simulink model "vehicle_hostmodel_2022b_v10"  (R2024b)
settings: Solver=ode4  StartTime=0.0  StopTime=inf  FixedStep=0.01  MaxStep=0.05  RelTol=1e-3
PreLoadFcn:
  | load("FInalGraph.mat")
model workspace (MAT data in the model file):
  G_final : digraph (value not decoded)
values from neighbouring files (symbols this model uses):
  ActorID = 0    [HelperSpeedActionAdapter.m]
  D = cross(B-A,C-A)    [HelperCalculateEgoRefPathInfo.m]
  L = zeros(N,1)    [HelperCalculateEgoRefPathInfo.m]
  psi_o = -1.185    [sensor.m]
  R = NaN(N,1)    [HelperCalculateEgoRefPathInfo.m]
  SceneInfo = [-32.1351766513 25.1612903226 -74.2242703533 -71.4592933948 -32.2887864823 26.2365591398 26.8509984639 27.0046082949 -32.7496159754 -72.380952381 -49.846390169 -49.3855606759 ... (30 elements, 10x3)]    [SceneLabels.mat]
  Ts = 0.05    [sensor.m]
undefined symbols (not defined in the file or in its folder): Acceleration, AngularVelocity, barrier_1, barrier_2, barrier_3, curvature, DefaultGear, DEND_B, DEND_S, DEND_T, direction, DiscIntNeverNeededParam, driving, finalint, goal1_coordinates, goal2_coordinates, goal3_coordinates, gradbp, latlongcoordinates, LF, LR, matlabshared, MAX_BRAKE, MAX_STEER, MAX_TORQUE, MCAR, MIN_BRAKE, MIN_STEER, MIN_TORQUE, NUMD_B, NUMD_S, NUMD_T, Pitch, Position, Roll, RRdamp, session, sigbuilder_block, STEER_RATIO, stopSign_ID, Tdead, thetaRefs, TL_ID, TrackWidth, ts, Vdead, Velocity, WB, xRef2s, Yaw, yRef2s
libraries: simulink x12, drivingscenarioandsensors x8, simulink_extras x5, drivingvehiclecontroller x2, trackingutilitieslib x2, robotalgslib x1, mpcadaslib x1, slpidlib x1, drivinglib x1, mpclib x1, autolibshared x1, vehdynlibviscommon x1
(part 1 of 4)
settings Model: SILPILSystemUnderTest=refmodels  Creator=akshran  LastModifiedBy=karto
settings DataIOCC: SignalLogging=off
settings OptimizationCC: ReuseModelBlockBuffer=off  ZeroExternalMemoryAtStartup=off  ZeroInternalMemoryAtStartup=off
settings DebuggingCC: UnconnectedInputMsg=warning  UnconnectedOutputMsg=warning  UnconnectedLineMsg=warning  UnderSpecifiedDimensionMsg=warning
settings HardwareCC: ProdBitPerLong=64  ProdHWDeviceType=Apple->ARM64
settings ModelReferenceCC: EnableRefExpFcnMdlSchedulingChecks=on
settings RTWCC: GenCodeOnly=on  TargetLang=C++  GPUComputeCapability=3.5  DLArmComputeVersion=19.05
settings GRTTargetCC: TargetLangStandard=C++11 (ISO)  MatFileLogging=off  CodeInterfacePackaging=C++ class

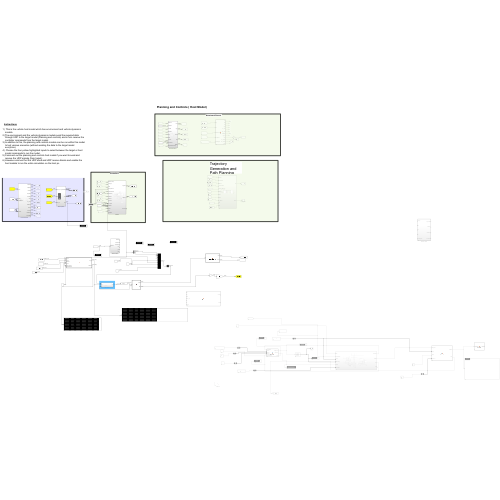
[thumbnail: Simulink's stored preview of the top-level diagram]
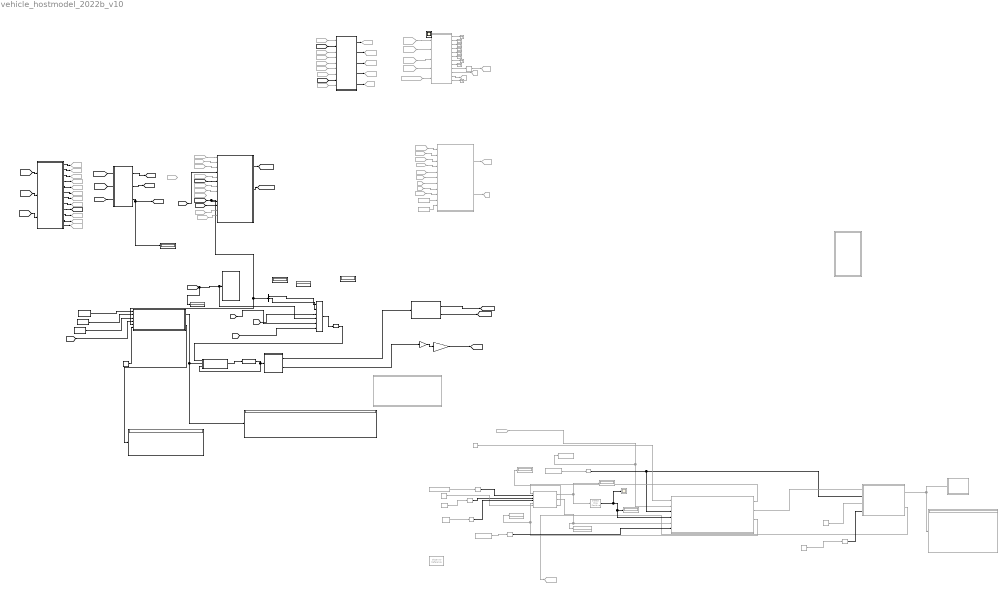
== system vehicle_hostmodel_2022b_v10 ==
  note: Trajectory Generation and Path Planning
  note: Trajectory Generation
  note: Behavioural Planner
  note: Instructions
      |
      | This is the vehicle host model which has environment and vehicle dynamics models.
      | The environment and the vehicle dynamics models send the required data through UDP to the target model (Planning and controls) and in turn receive the controller commands from the target model.
      | In addition to this, the planning and controls module can be run within this model to test various scenarios (without sending the data to the target model everytime).
      | Choose the four yellow highlighted inputs to select between the target or host model commands to run the model.
      | Comment out the planning and controls host model if you want to send and receive the UDP signals (from target).
      | Likewise comment out the UDP send and UDP receive blocks and enable the host models to run the entire simulation on the host pc.
  note: Environment & Vehicle Dynamics(Common Model)
  note: Planning and Controls ( Host Model)
  note: Controllers
  Behavioural Planner : Subsystem
  Constant : Constant  Value=xRef2s
  Constant1 : Constant  Commented=on  Value=latlongcoordinates
  Constant10 : Constant  Value=yRef2s
  Constant11 : Constant  Value=curvature
  Constant12 : Constant  Value=10
  Constant2 : Constant  Commented=on  Value=[latlongcoordinates(1,1) latlongcoordinates(1,2) 234]
  Constant3 : Constant  Commented=on  Value=barrier_1
  Constant4 : Constant  Commented=on  Value=40
  Constant5 : Constant  Commented=on  Value=234
  Constant6 : Constant  Commented=on  Value=goal1_coordinates
  Constant7 : Constant  Commented=on  Value=barrier_2
  Constant8 : Constant  Commented=on  Value=goal3_coordinates
  Constant9 : Constant  Commented=on  Value=barrier_3
  Controllers : Subsystem
  Demux : Demux  Outputs=3
  Detect Rise Positive : simulink/Logic and Bit Operations/Detect Rise Positive  Commented=through  vinit=0  OutDataTypeStr=boolean
  Display{,1..5} (6 alike) : Display  Commented=on
  Display{7..12,14} (7 alike) : Display
  Environment & Data : Subsystem
  From Workspace : FromWorkspace  Commented=on  VariableName=xRef2
  From Workspace1 : FromWorkspace  Commented=on  VariableName=yRef2
  From1 : From  Commented=on  GotoTag=CurrPos  TagVisibility=global
  From19 : From  Commented=on  GotoTag=obj_ahead  TagVisibility=global
  From21 : From  Commented=on  GotoTag=sceneID  TagVisibility=global
  From22 : From  Commented=on  GotoTag=objDist  TagVisibility=global
  From23 : From  Commented=on  GotoTag=D2S  TagVisibility=global
  From24 : From  Commented=on  GotoTag=SDist  TagVisibility=global
  From25 : From  Commented=on  GotoTag=TL_poses  TagVisibility=global
  From27 : From  Commented=on  GotoTag=obj_rel_vel  TagVisibility=global
  From28 : From  Commented=on  GotoTag=obj_rel_vel  TagVisibility=global
  From29 : From  Commented=on  GotoTag=RelDistMin  TagVisibility=global
  From31 : From  Commented=on  GotoTag=RefPoses
  From32 : From  Commented=on  GotoTag=direction
  From33 : From  Commented=on  GotoTag=curvature
  From36 : From  Commented=on  GotoTag=actorsInfo  TagVisibility=global
  From37 : From  Commented=on  GotoTag=ego_states  TagVisibility=global
  From38 : From  Commented=on  GotoTag=LaneBounds  TagVisibility=global
  From39 : From  Commented=on  GotoTag=RoadSpeed  TagVisibility=global
  From40 : From  Commented=on  GotoTag=CurrPos  TagVisibility=global
  From41 : From  Commented=on  GotoTag=curvature
  From42 : From  Commented=on  GotoTag=ego_vel  TagVisibility=global
  From43 : From  Commented=on  GotoTag=PositionMIO  TagVisibility=global
  From44 : From  Commented=on  GotoTag=obj_rel_vel  TagVisibility=global
  From45 : From  Commented=on  GotoTag=flagLC  TagVisibility=global
  From46 : From  Commented=on  GotoTag=laneL  TagVisibility=global
  From47 : From  Commented=on  GotoTag=desiredV  TagVisibility=global
  From48 : From  Commented=on  GotoTag=desiredV  TagVisibility=global
  From49 : From  Commented=on  GotoTag=laneR  TagVisibility=global
  From52 : From  Commented=on  GotoTag=Brake  TagVisibility=global
  From54 : From  Commented=on  GotoTag=Tgap  TagVisibility=global
  From55 : From  Commented=on  GotoTag=flagACC  TagVisibility=global
  From56 : From  Commented=on  GotoTag=LCinProgress  TagVisibility=global
  From58 : From  Commented=on  GotoTag=Acc  TagVisibility=global
  Gain1 : Gain  Gain=1/STEER_RATIO
  Gain2 : Gain  Gain=180/pi
  Goto1 : Goto  Commented=on  GotoTag=dest1  TagVisibility=global
  Goto10 : Goto  Commented=on  GotoTag=objDist  TagVisibility=global
  Goto11 : Goto  Commented=on  GotoTag=SDist  TagVisibility=global
  Goto12 : Goto  Commented=on  GotoTag=D2S  TagVisibility=global
  Goto13 : Goto  Commented=on  GotoTag=TL_poses  TagVisibility=global
  Goto16 : Goto  Commented=on  GotoTag=actorsInfo  TagVisibility=global
  Goto17 : Goto  Commented=on  GotoTag=RelDistMin  TagVisibility=global
  Goto21 : Goto  Commented=on  GotoTag=waypoints  TagVisibility=global
  Goto24 : Goto  Commented=on  GotoTag=trans_host  TagVisibility=global
  Goto25 : Goto  Commented=on  GotoTag=LaneBounds  TagVisibility=global
  Goto26 : Goto  Commented=on  GotoTag=PositionMIO  TagVisibility=global
  Goto27 : Goto  Commented=on  GotoTag=flagLC  TagVisibility=global
  Goto28 : Goto  Commented=on  GotoTag=desiredV  TagVisibility=global
  Goto29 : Goto  Commented=on  GotoTag=laneL  TagVisibility=global
  Goto30 : Goto  Commented=on  GotoTag=laneR  TagVisibility=global
  Goto32 : Goto  Commented=on  GotoTag=Brake  TagVisibility=global
  Goto33 : Goto  Commented=on  GotoTag=Tgap  TagVisibility=global
  Goto34 : Goto  Commented=on  GotoTag=flagACC  TagVisibility=global
  Goto6 : Goto  Commented=on  GotoTag=obj_ahead  TagVisibility=global
  Goto8 : Goto  Commented=on  GotoTag=obj_rel_vel  TagVisibility=global
  Goto9 : Goto  Commented=on  GotoTag=sceneID  TagVisibility=global
  LC_Progress : Goto  Commented=on  GotoTag=LC_ACC  TagVisibility=global
  MATLAB Function : MATLAB Function  Commented=on  TreatAsAtomicUnit=on
  MATLAB Function1 : MATLAB Function  Commented=through  TreatAsAtomicUnit=on
  MATLAB Function2 : MATLAB Function  TreatAsAtomicUnit=on
  MATLAB Function3 : MATLAB Function  Commented=on  TreatAsAtomicUnit=on
  MATLAB Function4 : MATLAB Function  Commented=on  TreatAsAtomicUnit=on
  MATLAB Function5 : MATLAB Function  Commented=on  TreatAsAtomicUnit=on
  MATLAB Function6 : MATLAB Function  TreatAsAtomicUnit=on
  MATLAB Function7 : MATLAB Function  TreatAsAtomicUnit=on
  Mux : Mux  Inputs=6
  NOT : Logic  Commented=on  Operator=NOT  IconShape=distinctive  AllPortsSameDT=off  OutDataTypeStr=boolean
  Observer : ObserverReference  Commented=on  ObserverModelName=vehicle_hostmodel_2022b_v10_Observer1
  Reference Data : Subsystem  VariantControl=Stanley
  Reference Data1 : Subsystem  Commented=on  TreatAsAtomicUnit=on  VariantControl=Stanley
  Reshape{,1..4,6} (6 alike) : Reshape  Commented=through  OutputDimensionality=Row vector (2-D)
  Reshape5 : Reshape  OutputDimensionality=Column vector (2-D)
  Scope2 : Scope  Commented=on
  Signal Specification : SignalSpecification  Dimensions=[2 1]
  Subsystem : Subsystem  Commented=on
  Subsystem2 : Subsystem  Commented=on
  Subsystem3 : Subsystem
  Terminator{,1..8} (9 alike) : Terminator  Commented=on
  To Workspace : ToWorkspace  Commented=on  VariableName=VehiclePos  SaveFormat=Timeseries  SampleTime=-1
  Vehicle Dynamics : Subsystem
  Scope : Scope
  Scope1 : Scope
  tag scope: CurrPos=global, MPCaccel=global, MPCdecel=global, VehInfo=global, brake_host=global, ego_states=global, ego_vel=global, steer_host=global, torque_host=global
  wires:
  Controllers/1(TorgueCm) -> [torque_host]
  Environment & Data/1(ObjAhead) -> Goto6/1
  Environment & Data/2(ObjRelVel) -> Goto8/1
  Environment & Data/3(SceneID) -> Goto9/1
  Environment & Data/4(ObjectDist) -> Goto10/1
  Environment & Data/6(SDist) -> Goto11/1
  Environment & Data/5(SceneDist) -> Goto12/1
  Environment & Data/7(TL_poses) -> Goto13/1
  Vehicle Dynamics/1(EgoVehStates) -> [ego_states]
  Vehicle Dynamics/3(xdot) -> Display8/1, [ego_vel]
  Environment & Data/8(RelDistmin) -> Goto17/1
  Vehicle Dynamics/2(Info) -> [VehInfo]
  [torque_host] -> Vehicle Dynamics/1(torque_cm)
  [brake_host] -> Vehicle Dynamics/2(brake_cm)
  [steer_host] -> Vehicle Dynamics/3(steer_cm)
  [trans_host] -> Environment & Data/1(Trans)
  [ego_states] -> Environment & Data/2(EgoVehStates)
  From28/1 -> Controllers/1(Relative velocity)
  From29/1 -> Controllers/5(Relative distance)
  [ego_vel] -> Controllers/6(CurrVelocity)
  From31/1 -> Controllers/7(RefPoses)
  From32/1 -> Controllers/8(Direction)
  [CurrPos] -> MATLAB Function2/5(current_position), Demux/1, Controllers/10(curr poses)
  [VehInfo] -> Environment & Data/3(VehFdbk)
  Environment & Data/9(CurrPos) -> [CurrPos]
  Environment & Data/10(actorsinfo) -> Goto16/1
  From37/1 -> MATLAB Function/1(ego)
  From36/1 -> MATLAB Function/2(act)
  Environment & Data/11(LaneBounds) -> Goto25/1
  From38/1 -> MATLAB Function/3(LaneBounds)
  From39/1 -> MATLAB Function/4(RoadSpeed)
  MATLAB Function/9(stay) -> NOT/1
  MATLAB Function/10(LL_Change) -> Goto29/1
  MATLAB Function/11(RL_Change) -> Goto30/1
  Environment & Data/12(PositionMIO) -> Goto26/1
  NOT/1 -> Goto27/1
  From54/1 -> Controllers/2(Time gap)
  From55/1 -> Controllers/3(ACC)
  From56/1 -> MATLAB Function/5(LCinProgress)
  [VehInfo] -> Controllers/11(VehFdbk)
  Controllers/2(BrakeCm) -> [brake_host]
  From45/1 -> Subsystem/1(function)
  From40/1 -> Subsystem/2(CurrentPose)
  From43/1 -> Subsystem/3(MIOPos)
  From41/1 -> Subsystem/4(Road Curvature)
  From42/1 -> Subsystem/5(Velocity_Initial_Ego)
  From44/1 -> Subsystem/6(MIOVel)
  From48/1 -> Subsystem/9(V_desired)
  Subsystem/2(check) -> LC_Progress/1
  From19/1 -> Behavioural Planner/1(ObjAhead)
  [ego_vel] -> Behavioural Planner/2(EgoSpeed)
  From21/1 -> Behavioural Planner/3(SceneID)
  From22/1 -> Behavioural Planner/4(ObjectDist)
  From23/1 -> Behavioural Planner/5(D2S)
  From24/1 -> Behavioural Planner/6(SDist)
  From25/1 -> Behavioural Planner/7(TLposes)
  [CurrPos] -> Behavioural Planner/8(CurrentPose)
  From27/1 -> Behavioural Planner/9(Object Relative Velocity)
  Behavioural Planner/1(Trans) -> Goto24/1
  Behavioural Planner/2(Tgap) -> Goto33/1
  Behavioural Planner/3(VelCmd) -> Goto28/1
  Behavioural Planner/4(ACC) -> Goto34/1
  Behavioural Planner/5(Braking) -> Goto32/1
  From52/1 -> Controllers/12(Brake)
  From58/1 -> Controllers/13(Acc)
  Subsystem/1(out) -> Goto21/1
  From46/1 -> Subsystem/7(laneL)
  From49/1 -> Subsystem/8(laneR)
  From Workspace/1 -> Subsystem/10(xref)
  From Workspace1/1 -> Subsystem/11(yref)
  MATLAB Function/1(ttc) -> Terminator/1
  MATLAB Function/2(dist) -> Terminator1/1
  MATLAB Function/3(left) -> Terminator2/1
  MATLAB Function/4(right) -> Terminator3/1
  MATLAB Function/5(LL_avail) -> Terminator4/1
  MATLAB Function/6(RL_avail) -> Terminator5/1
  MATLAB Function/7(tend2stay) -> Terminator6/1
  MATLAB Function/8(ego_vel) -> Terminator7/1
  MATLAB Function/12(y_lane) -> Terminator8/1
  [RoadSpeed] -> Controllers/4(velocity desired)
  From1/1 -> Subsystem2/2(CurrentPose), To Workspace/1
  MATLAB Function3/2(outbarrier) -> Display1/1, Subsystem2/5(barrier)
  MATLAB Function4/1(WPENU) -> Display/1, MATLAB Function1/1(EgoWayPts)
  MATLAB Function4/2(dest) -> Goto1/1
  Constant3/1 -> Reshape1/1
  Constant7/1 -> Reshape3/1
  Reshape3/1 -> MATLAB Function3/3(barrier2)
  Reshape/1 -> MATLAB Function4/2(origin), Subsystem2/3(origin)
  Constant4/1 -> MATLAB Function3/6(distanceBarrier)
  Subsystem2/3(flag) -> MATLAB Function3/5(ChkPointFlag), Display2/1
  Reshape1/1 -> MATLAB Function3/2(barrier1)
  Subsystem2/1(CurrPosLL) -> MATLAB Function3/1(CurrentPose)
  Constant1/1 -> Subsystem2/1(WP)
  MATLAB Function3/1(FlagBarrier) -> Detect Rise Positive/1, Display3/1
  Constant5/1 -> MATLAB Function4/3(height)
  Constant2/1 -> Reshape/1
  Reshape4/1 -> MATLAB Function4/4(goalcoord)
  Subsystem2/2(OutWP) -> MATLAB Function4/1(Waypoints)
  Reshape6/1 -> MATLAB Function3/4(barrier3)
  MATLAB Function3/3(dist) -> Display5/1
  Constant8/1 -> Reshape4/1
  Detect Rise Positive/1 -> Scope2/1, Subsystem2/4(BarrierFlag), Display4/1
  Constant6/1 -> Reshape2/1
  Reshape2/1 -> Subsystem2/6(checkpoint)
  Constant9/1 -> Reshape6/1
  Constant/1 -> MATLAB Function2/1(x_path)
  Constant10/1 -> MATLAB Function2/2(y_path)
  Constant11/1 -> MATLAB Function2/3(curvature)
  [RoadSpeed] -> MATLAB Function2/4(v_max)
  MATLAB Function2/1(ref_traj) -> Display12/1, Subsystem3/2(ref)
  [ego_vel] -> Display10/1, Mux/4, Reference Data/1(VelFdbk)
  [yawrate] -> Mux/6
  [ydot] -> Mux/5
  MATLAB Function7/2(steer) -> Gain2/1
  Gain2/1 -> Gain1/1
  Gain1/1 -> [steer_host]
  MATLAB Function7/1(throttle) -> MATLAB Function6/1(u)
  MATLAB Function6/1(accel) -> [MPCaccel]
  MATLAB Function6/2(deccel) -> [MPCdecel]
  Demux/1 -> Mux/1
  Demux/2 -> Mux/2
  [psi] -> Mux/3
  Mux/1 -> Reshape5/1
  Constant12/1 -> MATLAB Function2/6(PredictionHorizon)
  Signal Specification/1 -> MATLAB Function7/1(u), Subsystem3/3(In3)
  MATLAB Function2/2(distances) -> Display14/1
  Reshape5/1 -> Subsystem3/1(x)
  Subsystem3/1(mv) -> Signal Specification/1

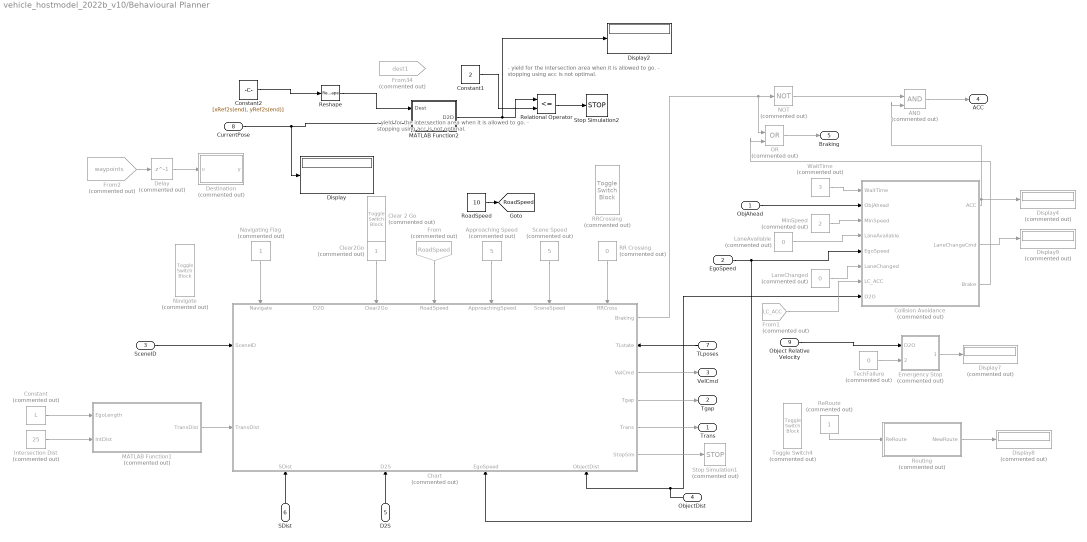
== system vehicle_hostmodel_2022b_v10/Behavioural Planner ==
  note: - yield for the intersection area when it is allowed to go.
      | - stopping using acc is not optimal.
  note: - yield for the intersection area when it is allowed to go.
      | - stopping using acc is not optimal.
  ObjAhead : Inport
  EgoSpeed : Inport  Port=2
  SceneID : Inport  Port=3
  ObjectDist : Inport  Port=4
  D2S : Inport  Port=5
  SDist : Inport  Port=6
  TLposes : Inport  Port=7
  CurrentPose : Inport  Port=8
  Object Relative Velocity : Inport  Port=9
  AND : Logic  Commented=on  IconShape=distinctive  AllPortsSameDT=off  OutDataTypeStr=fixdt(1,16)
  Approaching Speed : Constant  Commented=on  Value=5
  Chart : Stateflow chart  Commented=on  TreatAsAtomicUnit=on
      settings: PortSchema="{\"entries\":[{\"content\":{\"sides\":[{\"content\":{\"connectorIds\":[\"In14\",\"In2\"]},\"type\":\"ConnectorPlacement.EquallySpacedRectSide\",\"uuid\":\"81aca70f-0947-49fb-b60a-be241e44193b\"},{\"content\":{\"connectorIds\":[\"Out5\",\"In1\",\"Out1\",\"Out2\",\"Out3\",\"Out4\"],\"side\":\"RIGHT\"},\"type\":\"ConnectorPlacement.EquallySpacedRectSide\",\"uuid\":\"e7b9645e-3711-4964-ac9b-0199dd335e99\"},{\"content\":{\"connectorIds\":[\"In10\",\"In11\",\"In12\",\"In13\",\"In3\",\"In6\",\"In8\"],\"side\":\"TOP\"},\"type\":\"ConnectorPlacement.EquallySpacedRectSide\",\"uuid\":\"6876f024-944b-4540-9404-d68f37763657\"},{\"content\":{\"connectorIds\":[\"In7\",\"In9\",\"In4\",\"In5\"],\"side\":\"BOTTOM\"},\"type\":\"ConnectorPlacement.EquallySpacedRectSide\",\"uuid\":\"44acab73-cdde-4edf-95df-27422644ccab\"}]},\"type\":\"ConnectorPlacement.EquallySpacedConnector\",\"uuid\":\"d2c31c01-e447-43db-8d2b-8b98a0ca291a\"}],\"packageUris\":[\"http://schema.mathworks.com/mf0/Connector/R2020b\"],\"version\":\"1.0\"}"
  Clear 2 Go : ToggleSwitchBlock  Commented=on
      settings: Values={{'Off', 'On'}, [0 1]}
  Clear2Go : Constant  Commented=on
  Collision Avoidance : Stateflow chart  Commented=on  TreatAsAtomicUnit=on
  Constant : Constant  Commented=on  Value=L
  Constant1 : Constant  Value=2
  Constant2 : Constant  Value=[xRef2s(end), yRef2s(end)]
  Delay : Delay  Commented=on  DelayLength=1
  Destination : MATLAB Function  Commented=on  TreatAsAtomicUnit=on
  Display : Display
  Display2 : Display
  Display{4,7..9} (4 alike) : Display  Commented=on
  Emergency Stop : Stateflow chart  Commented=on  TreatAsAtomicUnit=on
  From : From  Commented=on  GotoTag=RoadSpeed  TagVisibility=global
  From1 : From  Commented=on  GotoTag=LC_ACC
  From2 : From  Commented=on  GotoTag=waypoints  TagVisibility=global
  From34 : From  Commented=on  GotoTag=dest1
  Intersection Dist : Constant  Commented=on  Value=25
  LaneAvailable : Constant  Commented=on  Value=0
  LaneChanged : Constant  Commented=on  Value=0
  MATLAB Function1 : MATLAB Function  Commented=on  TreatAsAtomicUnit=on
  MATLAB Function2 : MATLAB Function  TreatAsAtomicUnit=on
  MinSpeed : Constant  Commented=on  Value=2
  NOT : Logic  Commented=on  Operator=NOT  IconShape=distinctive  AllPortsSameDT=off  OutDataTypeStr=boolean
  Navigate : ToggleSwitchBlock  Commented=on
      settings: Values={{'Off', 'On'}, [0 1]}
  Navigating Flag : Constant  Commented=on
  OR : Logic  Commented=on  Operator=OR  IconShape=distinctive  AllPortsSameDT=off  OutDataTypeStr=boolean
  RR Crossing : Constant  Commented=on  Value=0
  RRCrossing : ToggleSwitchBlock  Commented=on
      settings: Values={{'Off', 'On'}, [0 1]}
  ReRoute : Constant  Commented=on
  Relational Operator : RelationalOperator  Operator=<=  OutDataTypeStr=boolean  RndMeth=Simplest  InputSameDT=off
  Reshape : Reshape  OutputDimensionality=Row vector (2-D)
  RoadSpeed : Constant  Value=10
  Routing : Stateflow chart  Commented=on  TreatAsAtomicUnit=on
  Scene Speed : Constant  Commented=on  Value=5
  Stop Simulation1 : Stop  Commented=on
  Stop Simulation2 : Stop
  TechFailure : Constant  Commented=on  Value=0
  Toggle Switch4 : ToggleSwitchBlock  Commented=on
      settings: Values={{'Off', 'On'}, [0 1]}
  WaitTime : Constant  Commented=on  Value=3
  Trans : Outport
  Tgap : Outport  Port=2
  VelCmd : Outport  Port=3
  ACC : Outport  Port=4
  Braking : Outport  Port=5
  tag scope: RoadSpeed=global
  wires:
  Clear2Go/1 -> Chart/12(Clear2Go)
  Routing/1(NewRoute) -> Display8/1
  ObjectDist/1 -> Chart/5(ObjectDist), Collision Avoidance/8(D2O)
  WaitTime/1 -> Collision Avoidance/1(WaitTime)
  Navigating Flag/1 -> Chart/10(Navigate)
  Approaching Speed/1 -> Chart/3(ApproachingSpeed)
  Scene Speed/1 -> Chart/6(SceneSpeed)
  EgoSpeed/1 -> Collision Avoidance/5(EgoSpeed), Chart/4(EgoSpeed)
  ReRoute/1 -> Routing/1(ReRoute)
  Collision Avoidance/2(LaneChangeCmd) -> Display9/1
  LaneAvailable/1 -> Collision Avoidance/4(LaneAvailable)
  RR Crossing/1 -> Chart/8(RRCross)
  MinSpeed/1 -> Collision Avoidance/3(MinSpeed)
  LaneChanged/1 -> Collision Avoidance/6(LaneChanged)
  From/1 -> Chart/13(RoadSpeed)
  ObjAhead/1 -> Collision Avoidance/2(ObjAhead)
  SceneID/1 -> Chart/14(SceneID)
  Chart/4(StopSim) -> Stop Simulation1/1
  Chart/3(Trans) -> Trans/1
  TLposes/1 -> Chart/1(TLstate)
  Chart/1(VelCmd) -> VelCmd/1
  SDist/1 -> Chart/7(SDist)
  D2S/1 -> Chart/9(D2S)
  Chart/2(Tgap) -> Tgap/1
  TechFailure/1 -> Emergency Stop/2(TechFailure)
  Emergency Stop/1(EStop) -> Display7/1
  Object Relative Velocity/1 -> Emergency Stop/1(D2O)
  Collision Avoidance/1(ACC) -> AND/2, Display4/1
  RoadSpeed/1 -> [RoadSpeed]
  NOT/1 -> AND/1
  AND/1 -> ACC/1
  Chart/5(Braking) -> OR/1, NOT/1
  OR/1 -> Braking/1
  Collision Avoidance/3(Brake) -> OR/2
  Constant/1 -> MATLAB Function1/1(EgoLength)
  Intersection Dist/1 -> MATLAB Function1/2(IntDist)
  MATLAB Function1/1(TransDist) -> Chart/2(TransDist)
  From1/1 -> Collision Avoidance/7(LC_ACC)
  From2/1 -> Delay/1
  Delay/1 -> Destination/1(u)
  CurrentPose/1 -> Display/1, MATLAB Function2/2(CurrentPose)
  Relational Operator/1 -> Stop Simulation2/1
  Constant1/1 -> Relational Operator/2
  MATLAB Function2/1(D2D) -> Display2/1, Relational Operator/1
  Constant2/1 -> Reshape/1
  Reshape/1 -> MATLAB Function2/1(Dest)

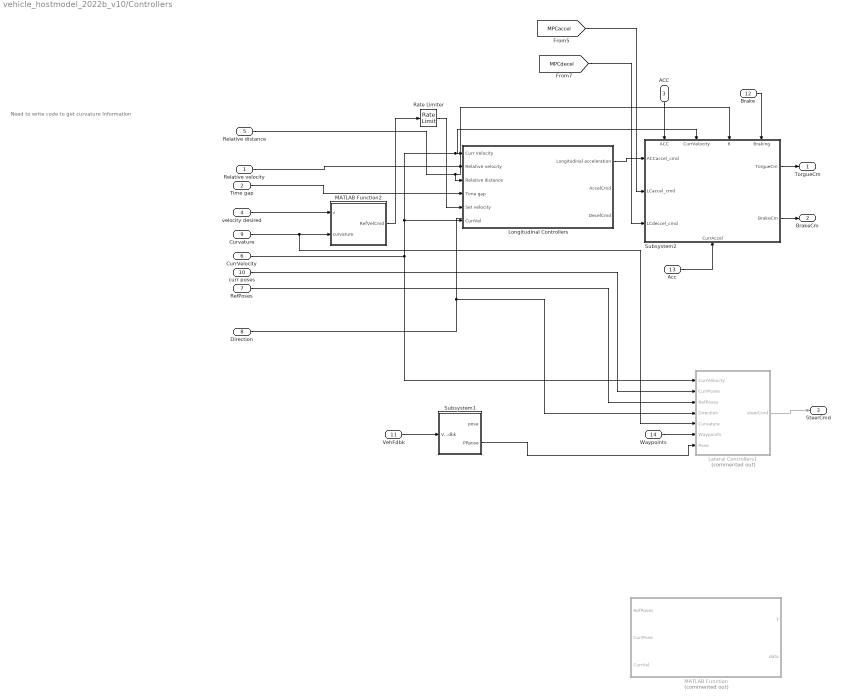
== system vehicle_hostmodel_2022b_v10/Controllers ==
  note: Need to write code to get curvature Information
  Relative velocity : Inport
  Time gap : Inport  Port=2
  ACC : Inport  Port=3
  velocity desired : Inport  Port=4
  Relative distance : Inport  Port=5
  CurrVelocity : Inport  Port=6
  RefPoses : Inport  Port=7
  Direction : Inport  Port=8
  Curvature : Inport  Port=9
  curr poses : Inport  Port=10
  VehFdbk : Inport  Port=11
  Brake : Inport  Port=12
  Acc : Inport  Port=13
  Waypoints : Inport  Port=14
  Lateral Controllers1 : Subsystem  Commented=on
  Longitudinal Controllers : Subsystem
  MATLAB Function : MATLAB Function  Commented=on  TreatAsAtomicUnit=on
  MATLAB Function2 : MATLAB Function  TreatAsAtomicUnit=on
  Rate Limiter : RateLimiter  RisingSlewLimit=2  SampleTimeMode=inherited
  Subsystem1 : Subsystem
  Subsystem2 : Subsystem
      settings: PortSchema="{\"entries\":[{\"content\":{\"sides\":[{\"content\":{\"connectorIds\":[\"In1\",\"In2\",\"In3\"]},\"type\":\"ConnectorPlacement.EquallySpacedRectSide\",\"uuid\":\"a23b1a10-3bcb-40a0-900c-c9a3f160b173\"},{\"content\":{\"connectorIds\":[\"Out1\",\"Out2\"],\"side\":\"RIGHT\"},\"type\":\"ConnectorPlacement.EquallySpacedRectSide\",\"uuid\":\"88840b66-912f-4184-aeec-297642319416\"},{\"content\":{\"connectorIds\":[\"In4\",\"In5\",\"In6\",\"In7\"],\"side\":\"TOP\"},\"type\":\"ConnectorPlacement.EquallySpacedRectSide\",\"uuid\":\"37a03ca9-b065-473e-b290-3b07703c6005\"},{\"content\":{\"connectorIds\":[\"In8\"],\"side\":\"BOTTOM\"},\"type\":\"ConnectorPlacement.EquallySpacedRectSide\",\"uuid\":\"275ca825-7815-497a-af18-67b3ec4705b4\"}]},\"type\":\"ConnectorPlacement.EquallySpacedConnector\",\"uuid\":\"5bfc7c71-8f7a-4cba-a168-7eeca22a2fcb\"}],\"packageUris\":[\"http://schema.mathworks.com/mf0/Connector/R2020b\"],\"version\":\"1.0\"}"
  TorgueCm : Outport
  BrakeCm : Outport  Port=2
  SteerCmd : Outport  Port=3
  wires:
  Curvature/1 -> MATLAB Function2/2(curvature), Lateral Controllers1/5(Curvature)
  Relative velocity/1 -> Longitudinal Controllers/2(Relative velocity)
  Direction/1 -> Lateral Controllers1/4(Direction)
  RefPoses/1 -> Lateral Controllers1/3(RefPoses)
  velocity desired/1 -> MATLAB Function2/1(v)
  CurrVelocity/1 -> Subsystem2/5(CurrVelocity), Longitudinal Controllers/1(Curr Velocity), Longitudinal Controllers/6(CurrVel), Lateral Controllers1/1(CurrVelocity)
  Time gap/1 -> Longitudinal Controllers/4(Time gap)
  Relative distance/1 -> Subsystem2/6(Relative Distance), Longitudinal Controllers/3(Relative distance)
  Subsystem1/2(PPpose) -> Lateral Controllers1/7(Pose)
  VehFdbk/1 -> Subsystem1/1(VehFdbk)
  Lateral Controllers1/1(steerCmd) -> SteerCmd/1
  Rate Limiter/1 -> Longitudinal Controllers/5(Set velocity)
  curr poses/1 -> Lateral Controllers1/2(CurrPoses)
  Longitudinal Controllers/1(Longitudinal acceleration) -> Subsystem2/1(ACCaccel_cmd)
  ACC/1 -> Subsystem2/4(ACC)
  Subsystem2/1(TorgueCm) -> TorgueCm/1
  Subsystem2/2(BrakeCm) -> BrakeCm/1
  Acc/1 -> Subsystem2/8(CurrAccel)
  Brake/1 -> Subsystem2/7(Braking)
  Waypoints/1 -> Lateral Controllers1/6(Waypoints)
  MATLAB Function2/1(RefVelCmd) -> Rate Limiter/1
  [MPCaccel] -> Subsystem2/2(LCaccel_cmd)
  [MPCdecel] -> Subsystem2/3(LCdeccel_cmd)

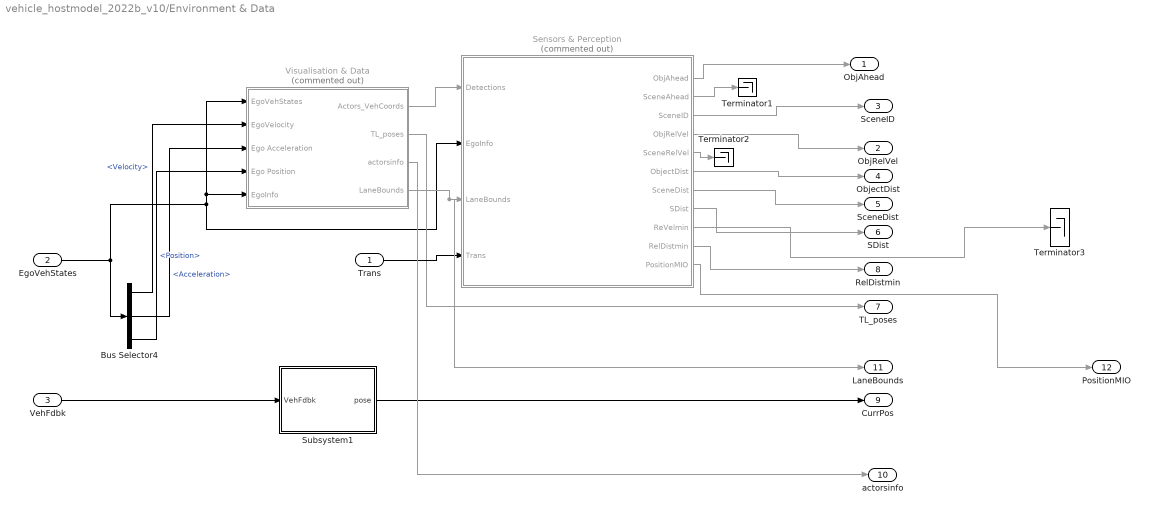
== system vehicle_hostmodel_2022b_v10/Environment & Data ==
  Trans : Inport
  EgoVehStates : Inport  Port=2
  VehFdbk : Inport  Port=3
  Bus Selector4 : BusSelector  OutputSignals=Velocity,Acceleration,Position
  Sensors & Perception : Subsystem  Commented=on
  Subsystem1 : Subsystem
  Terminator1 : Terminator
  Terminator2 : Terminator
  Terminator3 : Terminator
  Visualisation & Data : Subsystem  Commented=on
  ObjAhead : Outport
  ObjRelVel : Outport  Port=2
  SceneID : Outport  Port=3
  ObjectDist : Outport  Port=4
  SceneDist : Outport  Port=5
  SDist : Outport  Port=6
  TL_poses : Outport  Port=7
  RelDistmin : Outport  Port=8
  CurrPos : Outport  Port=9
  actorsinfo : Outport  Port=10
  LaneBounds : Outport  Port=11
  PositionMIO : Outport  Port=12
  wires:
  Bus Selector4/3 -> Visualisation & Data/4(Ego Position)  "<Position>"
  Sensors & Perception/1(ObjAhead) -> ObjAhead/1
  Bus Selector4/1 -> Visualisation & Data/2(EgoVelocity)  "<Velocity>"
  Visualisation & Data/1(Actors_VehCoords) -> Sensors & Perception/1(Detections)
  Sensors & Perception/5(SceneRelVel) -> Terminator2/1
  Sensors & Perception/2(SceneAhead) -> Terminator1/1
  Sensors & Perception/6(ObjectDist) -> ObjectDist/1
  Bus Selector4/2 -> Visualisation & Data/3(Ego Acceleration)  "<Acceleration>"
  Sensors & Perception/9(ReVelmin) -> Terminator3/1
  EgoVehStates/1 -> Visualisation & Data/5(EgoInfo), Visualisation & Data/1(EgoVehStates), Sensors & Perception/2(EgoInfo), Bus Selector4/1
  Sensors & Perception/4(ObjRelVel) -> ObjRelVel/1
  Visualisation & Data/2(TL_poses) -> TL_poses/1
  Sensors & Perception/3(SceneID) -> SceneID/1
  Sensors & Perception/8(SDist) -> SDist/1
  Sensors & Perception/7(SceneDist) -> SceneDist/1
  Trans/1 -> Sensors & Perception/4(Trans)
  Sensors & Perception/10(RelDistmin) -> RelDistmin/1
  VehFdbk/1 -> Subsystem1/1(VehFdbk)
  Subsystem1/1(pose) -> CurrPos/1
  Visualisation & Data/3(actorsinfo) -> actorsinfo/1
  Visualisation & Data/4(LaneBounds) -> LaneBounds/1, Sensors & Perception/3(LaneBounds)
  Sensors & Perception/11(PositionMIO) -> PositionMIO/1

== system vehicle_hostmodel_2022b_v10/Reference Data ==
  note: Select method to calculate theta
  VelFdbk : Inport
  Curvature : Lookup_n-D  NumberOfTableDimensions=1  BreakpointsForDimension1=gradbp  Table=curvature  InternalRulePriority=Speed  RndMeth=Simplest
  Direction : Lookup_n-D  NumberOfTableDimensions=1  BreakpointsForDimension1=gradbp  Table=direction  InternalRulePriority=Speed  RndMeth=Simplest
  Display : Display
  Display1 : Display
  Integrator : Integrator
  Mux : Mux  Inputs=3
  Theta : Subsystem  Variant=on  VariantControlMode=label  LabelModeActiveChoice=thetaSimulinkBlock
  To Workspace : ToWorkspace  VariableName=x  SaveFormat=Timeseries  SampleTime=-1
  To Workspace1 : ToWorkspace  VariableName=y  SaveFormat=Timeseries  SampleTime=-1
  X Ref : Lookup_n-D  NumberOfTableDimensions=1  BreakpointsForDimension1=gradbp  Table=xRef2s  InternalRulePriority=Speed  RndMeth=Simplest
  Y Ref : Lookup_n-D  NumberOfTableDimensions=1  BreakpointsForDimension1=gradbp  Table=yRef2s  InternalRulePriority=Speed  RndMeth=Simplest
  RefPose : Outport
  DirectionO : Outport  Port=2
  CurvatureO : Outport  Port=3
  xref : Outport  Port=4
  yref : Outport  Port=5
  yaw : Outport  Port=6
  tag scope: xRef=global, yRef=global
  wires:
  Direction/1 -> DirectionO/1
  Curvature/1 -> CurvatureO/1
  Y Ref/1 -> Theta/1(y), Mux/2, yref/1, To Workspace1/1, Display1/1, [yRef]
  Mux/1 -> RefPose/1
  X Ref/1 -> Display/1, To Workspace/1, xref/1, Theta/2(x), Mux/1, [xRef]
  Integrator/1 -> Curvature/1, Direction/1, Theta/3(dis), Y Ref/1, X Ref/1
  VelFdbk/1 -> Integrator/1
  Theta/1(theta) -> yaw/1, Mux/3

== system vehicle_hostmodel_2022b_v10/Reference Data1 ==
  velEgo : Inport
  xd : Inport  Port=2
  yd : Inport  Port=3
  In4 : Inport  Port=4
  LCinProgress : Inport  Port=5
  Discrete-Time Integrator : DiscreteIntegrator  SampleTime=-1  ICPrevOutput=DiscIntNeverNeededParam  ICPrevScaledInput=DiscIntNeverNeededParam
  Memory : Memory
  Memory1 : Memory
  Merge : Merge
  Merge1 : Merge
  Subsystem : Subsystem
  Subsystem1 : Subsystem
  Subsystem2 : Subsystem
  Subsystem3 : Subsystem
  Switch : Switch  Criteria=u2 ~= 0  SaturateOnIntegerOverflow=off  InputSameDT=off
  Switch Case : SwitchCase  CaseConditions={1,0}  ShowDefaultCase=off
  waypointPP : Outport
  RefPose : Outport  Port=2
  DirectionO : Outport  Port=3
  CurvatureO : Outport  Port=4
  wires:
  velEgo/1 -> Subsystem3/1(VelFdbk), Subsystem2/1(VelFdbk), Discrete-Time Integrator/1
  Subsystem2/4(WayPoints) -> Merge1/1
  Merge1/1 -> waypointPP/1
  Subsystem2/1(RefPose) -> Switch/3
  Subsystem2/2(DirectionO) -> DirectionO/1
  Merge/1 -> CurvatureO/1
  Subsystem2/3(CurvatureO) -> Merge/2
  Subsystem3/1(RefPose) -> Switch/1
  Switch Case/1 -> Subsystem3/Action
  Switch Case/2 -> Subsystem2/Action
  xd/1 -> Memory/1
  yd/1 -> Memory1/1
  Memory/1 -> Subsystem3/2(xd)
  Memory1/1 -> Subsystem3/4(yd)
  Subsystem2/5(finalint) -> Subsystem3/3(finalint)
  Subsystem/1(Out1) -> Switch/2, Switch Case/1, Subsystem1/2(enable)
  LCinProgress/1 -> Subsystem/Enable
  Discrete-Time Integrator/1 -> Subsystem1/1(Integrator)
  Subsystem1/1(Ref pose) -> RefPose/1

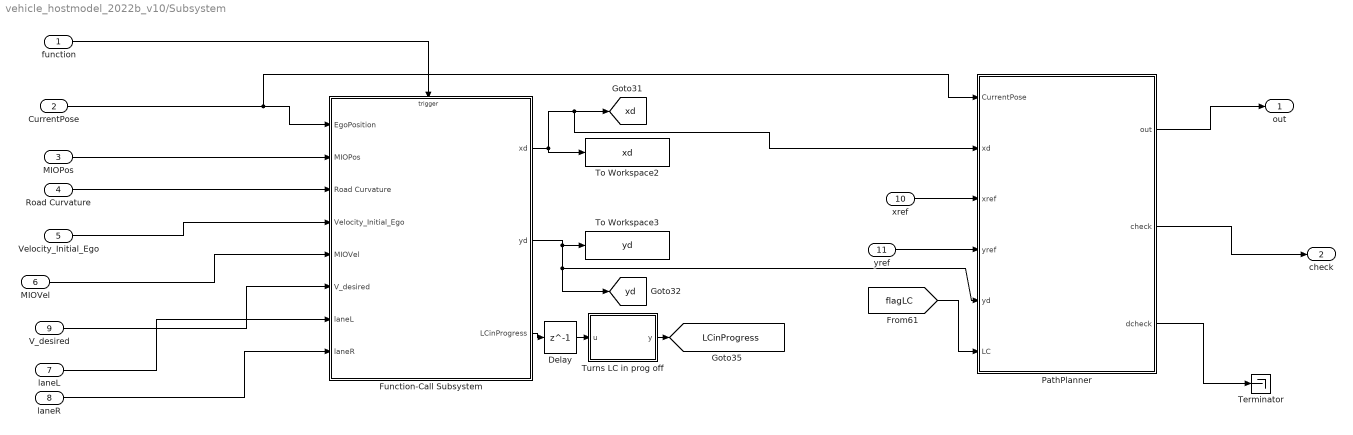
== system vehicle_hostmodel_2022b_v10/Subsystem ==
  function : Inport
  CurrentPose : Inport  Port=2
  MIOPos : Inport  Port=3
  Road Curvature : Inport  Port=4
  Velocity_Initial_Ego : Inport  Port=5
  MIOVel : Inport  Port=6
  laneL : Inport  Port=7
  laneR : Inport  Port=8
  V_desired : Inport  Port=9
  xref : Inport  Port=10
  yref : Inport  Port=11
  Delay : Delay  DelayLength=1
  Function-Call Subsystem : Subsystem  TreatAsAtomicUnit=on
  PathPlanner : Subsystem
  Terminator : Terminator
  To Workspace2 : ToWorkspace  VariableName=xd  SampleTime=-1
      settings: Save2DSignal=2-D array (concatenate along first dimension)
  To Workspace3 : ToWorkspace  VariableName=yd  SampleTime=-1
      settings: Save2DSignal=2-D array (concatenate along first dimension)
  Turns LC in prog off : MATLAB Function  TreatAsAtomicUnit=on
  out : Outport
  check : Outport  Port=2
  tag scope: LCinProgress=global, xd=global, yd=global
  wires:
  MIOVel/1 -> Function-Call Subsystem/5(MIOVel)
  Road Curvature/1 -> Function-Call Subsystem/3(Road Curvature)
  PathPlanner/1(out) -> out/1
  PathPlanner/2(check) -> check/1
  Velocity_Initial_Ego/1 -> Function-Call Subsystem/4(Velocity_Initial_Ego)
  V_desired/1 -> Function-Call Subsystem/6(V_desired)
  MIOPos/1 -> Function-Call Subsystem/2(MIOPos)
  Function-Call Subsystem/1(xd) -> To Workspace2/1, PathPlanner/2(xd), [xd]
  Function-Call Subsystem/2(yd) -> PathPlanner/5(yd), [yd], To Workspace3/1
  [flagLC] -> PathPlanner/6(LC)
  Delay/1 -> Turns LC in prog off/1(u)
  Turns LC in prog off/1(y) -> [LCinProgress]
  Function-Call Subsystem/3(LCinProgress) -> Delay/1
  CurrentPose/1 -> PathPlanner/1(CurrentPose), Function-Call Subsystem/1(EgoPosition)
  function/1 -> Function-Call Subsystem/Trigger
  laneL/1 -> Function-Call Subsystem/7(laneL)
  laneR/1 -> Function-Call Subsystem/8(laneR)
  xref/1 -> PathPlanner/3(xref)
  yref/1 -> PathPlanner/4(yref)
  PathPlanner/3(dcheck) -> Terminator/1

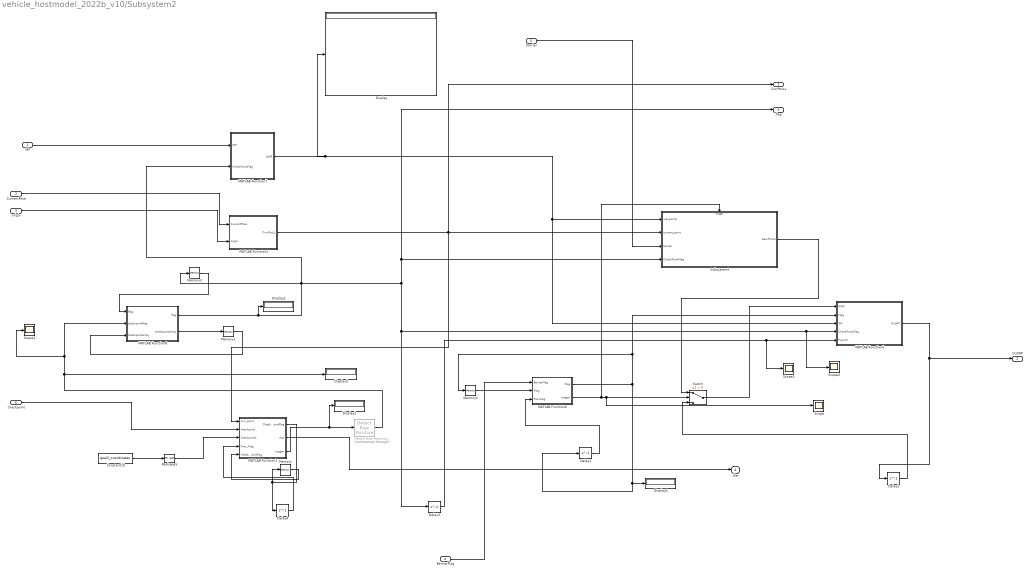
== system vehicle_hostmodel_2022b_v10/Subsystem2 ==
  WP : Inport
  CurrentPose : Inport  Port=2
  origin : Inport  Port=3
  BarrierFlag : Inport  Port=4
  barrier : Inport  Port=5
  checkpoint : Inport  Port=6
  Constant10 : Constant  Value=goal2_coordinates
  Delay{1..4} (4 alike) : Delay  DelayLength=1
  Detect Rise Positive1 : simulink/Logic and Bit Operations/Detect Rise Positive  Commented=through  vinit=0  OutDataTypeStr=boolean
  Display{,1..4} (5 alike) : Display
  MATLAB Function1 : MATLAB Function  TreatAsAtomicUnit=on
  MATLAB Function2 : MATLAB Function  TreatAsAtomicUnit=on
  MATLAB Function5 : MATLAB Function  TreatAsAtomicUnit=on
  MATLAB Function6 : MATLAB Function  TreatAsAtomicUnit=on
  MATLAB Function7 : MATLAB Function  TreatAsAtomicUnit=on
  MATLAB Function8 : MATLAB Function  TreatAsAtomicUnit=on
  Memory : Memory
  Memory1 : Memory  InitialCondition=zeros(1,2)
  Memory2 : Memory
  Memory3 : Memory
  Reshape5 : Reshape  OutputDimensionality=Row vector (2-D)
  Scope{,1..3} (4 alike) : Scope
  Subsystem1 : Subsystem
  Switch : Switch  Criteria=u2 > Threshold  SaturateOnIntegerOverflow=off  InputSameDT=off
  CurrPosLL : Outport
  OutWP : Outport  Port=2
  flag : Outport  Port=3
  dist : Outport  Port=4
  wires:
  Memory2/1 -> MATLAB Function6/2("Flag ")
  WP/1 -> MATLAB Function7/1(WP)
  Memory3/1 -> MATLAB Function8/1("flag ")
  Subsystem1/1(NewPoints) -> Switch/1
  Delay2/1 -> Switch/3
  barrier/1 -> Subsystem1/3(barrier)
  MATLAB Function2/1(CurrPosLL) -> Subsystem1/2(current_point), CurrPosLL/1, MATLAB Function1/1(curr_point)
  MATLAB Function8/1(flag) -> Display2/1, Subsystem1/4(CheckPointFlag), flag/1, Delay3/1, Scope3/1, MATLAB Function5/4(CheckPointFlag), Memory3/1, MATLAB Function7/2(CheckPointFlag)
  CurrentPose/1 -> MATLAB Function2/1(CurrentPose)
  Delay1/1 -> MATLAB Function6/3(PrevFlag)
  Memory1/1 -> MATLAB Function8/3("checkpointarray ")
  origin/1 -> MATLAB Function2/2(origin)
  MATLAB Function5/1(OutWP) -> Delay2/1, OutWP/1
  Delay3/1 -> Scope2/1, MATLAB Function5/5(PrevCF)
  BarrierFlag/1 -> MATLAB Function6/1(BarrierFlag)
  MATLAB Function6/2(trigger) -> Scope/1, Switch/2, Subsystem1/Trigger
  Detect Rise Positive1/1 -> Scope1/1, MATLAB Function8/2(checkpointflag), Display3/1
  MATLAB Function8/2(checkpointarray) -> Memory1/1
  MATLAB Function1/2(dist) -> dist/1
  MATLAB Function7/1(OWP) -> Display/1, MATLAB Function5/3(WP), Subsystem1/1(waypoints)
  Switch/1 -> MATLAB Function5/1(NWP)
  MATLAB Function6/1(Flag) -> Delay1/1, Display4/1, MATLAB Function5/2(Flag), Memory2/1
  checkpoint/1 -> MATLAB Function1/2(checkpoint)
  Constant10/1 -> Reshape5/1
  Reshape5/1 -> MATLAB Function1/3(checkpoint1)
  MATLAB Function1/3(trigger) -> Display1/1, Detect Rise Positive1/1
  MATLAB Function1/1(CheckPointFlag) -> Memory/1, Delay4/1
  Memory/1 -> MATLAB Function1/5("CheckPointFlag ")
  Delay4/1 -> MATLAB Function1/4(Prev_Flag)

== system vehicle_hostmodel_2022b_v10/Subsystem3 ==
  x : Inport
  ref : Inport  Port=2
  In3 : Inport  Port=3
  Delay : Delay  DelayLength=1  InitialCondition=0  UseCircularBuffer=on
  Subsystem1 : Subsystem  TreatAsAtomicUnit=on
  mv : Outport
  wires:
  In3/1 -> Delay/1
  Delay/1 -> Subsystem1/3(last_mv)
  x/1 -> Subsystem1/1(x)
  ref/1 -> Subsystem1/2(ref)
  Subsystem1/1(mv) -> mv/1

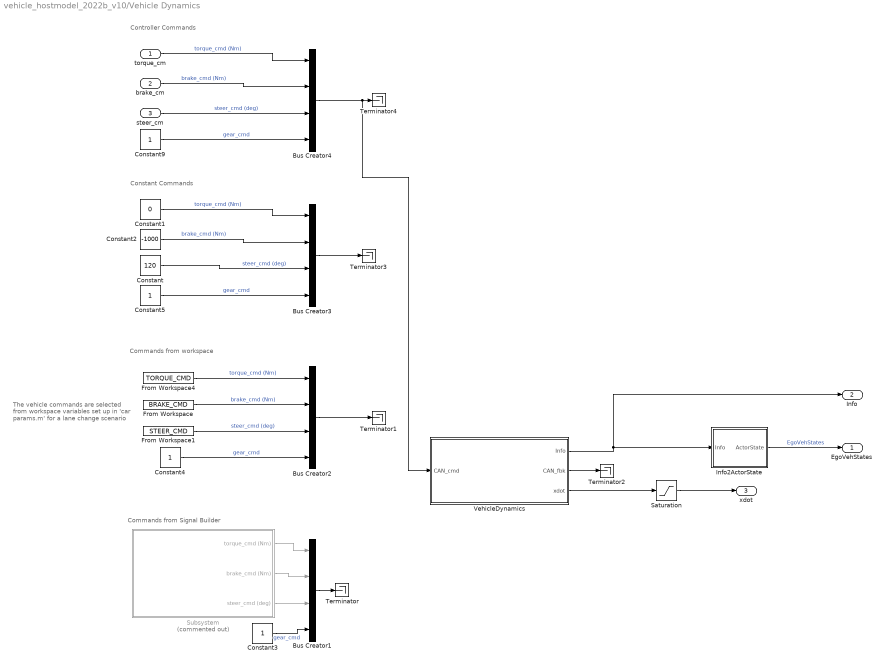
== system vehicle_hostmodel_2022b_v10/Vehicle Dynamics ==
  note: Constant Commands
  note: Commands from workspace
  note: Commands from Signal Builder
  note: The vehicle commands are selected from workspace variables set up in 'car params.m' for a lane change scenario
  note: Controller Commands
  torque_cm : Inport
  brake_cm : Inport  Port=2
  steer_cm : Inport  Port=3
  Bus Creator{1..4} (4 alike) : BusCreator  Inputs=4
  Constant : Constant  Value=120
  Constant1 : Constant  Value=0
  Constant2 : Constant  Value=-1000
  Constant{3..5,9} (4 alike) : Constant
  From Workspace : FromWorkspace  VariableName=BRAKE_CMD  SampleTime=ts
  From Workspace1 : FromWorkspace  VariableName=STEER_CMD  SampleTime=ts
  From Workspace4 : FromWorkspace  VariableName=TORQUE_CMD  SampleTime=ts
  Info2ActorState : Subsystem
  Saturation : Saturate  UpperLimit=inf  LowerLimit=0.001
  Subsystem : Subsystem  Commented=on
  Terminator{,1..4} (5 alike) : Terminator
  VehicleDynamics : Subsystem  mask{InitPosition=[xRef2s(1), yRef2s(1), 0], InitSpeed=0, InitYaw=0.009885}
      mask prompts: InitPosition "Initial Position (m)"; InitSpeed "Initial Speed (m/s)"; InitYaw "Init Yaw (rad)"
  EgoVehStates : Outport
  Info : Outport  Port=2
  xdot : Outport  Port=3
  wires:
  Bus Creator2/1 -> Terminator1/1
  VehicleDynamics/2(CAN_fbk) -> Terminator2/1
  VehicleDynamics/1(Info) -> Info/1, Info2ActorState/1(Info)
  Constant/1 -> Bus Creator3/3  "steer_cmd (deg)"
  Info2ActorState/1(ActorState) -> EgoVehStates/1  "EgoVehStates"
  Constant1/1 -> Bus Creator3/1  "torque_cmd (Nm)"
  Constant2/1 -> Bus Creator3/2  "brake_cmd (Nm)"
  VehicleDynamics/3(xdot) -> Saturation/1
  Subsystem/1(torque_cmd (Nm)) -> Bus Creator1/1
  Subsystem/2(brake_cmd (Nm)) -> Bus Creator1/2
  Subsystem/3(steer_cmd (deg)) -> Bus Creator1/3
  Constant3/1 -> Bus Creator1/4  "gear_cmd"
  Constant4/1 -> Bus Creator2/4  "gear_cmd"
  From Workspace/1 -> Bus Creator2/2  "brake_cmd (Nm)"
  From Workspace1/1 -> Bus Creator2/3  "steer_cmd (deg)"
  From Workspace4/1 -> Bus Creator2/1  "torque_cmd (Nm)"
  Constant5/1 -> Bus Creator3/4  "gear_cmd"
  Bus Creator1/1 -> Terminator/1
  brake_cm/1 -> Bus Creator4/2  "brake_cmd (Nm)"
  Constant9/1 -> Bus Creator4/4  "gear_cmd"
  torque_cm/1 -> Bus Creator4/1  "torque_cmd (Nm)"
  steer_cm/1 -> Bus Creator4/3  "steer_cmd (deg)"
  Bus Creator3/1 -> Terminator3/1
  Bus Creator4/1 -> VehicleDynamics/1(CAN_cmd), Terminator4/1
  Saturation/1 -> xdot/1

== system vehicle_hostmodel_2022b_v10/Controllers/Lateral Controllers1 ==
  note: include toggle logic
  CurrVelocity : Inport
  CurrPoses : Inport  Port=2
  RefPoses : Inport  Port=3
  Direction : Inport  Port=4
  Curvature : Inport  Port=5
  Waypoints : Inport  Port=6
  Pose : Inport  Port=7
  Constant : Constant  Commented=on
  Demux : Demux  Commented=on  Outputs=3
  Demux1 : Demux  Commented=on  Outputs=3
  From : From  Commented=on  GotoTag=yawrate  TagVisibility=global
  Gain : Gain  Gain=1/STEER_RATIO
  Gain1 : Gain  Commented=on  Gain=180/pi
  Gain2 : Gain  Gain=180/pi
  Lateral Controller Stanley : drivingvehiclecontroller/Lateral Controller Stanley  Commented=on  ModelType=Kinematic bicycle model  PositionGainF=0.75  PositionGainR=2.5  YawRateGain=0.05  DelayGain=0.05  VehicleMass=MCAR  Lf=LF  Lr=LR  TireStiffness=5e3  Wheelbase=3  MaxSteeringAngle=30
  Pure Pursuit Controller1 : Subsystem
  Scope2 : Scope  Commented=on  NumInputPorts=2
  Unit Delay : UnitDelay  Commented=on  SampleTime=-1  HasFrameUpgradeWarning=on
  steerCmd : Outport
  wires:
  From/1 -> Gain1/1
  CurrPoses/1 -> Demux1/1, Lateral Controller Stanley/2
  Pure Pursuit Controller1/1(delta) -> Gain2/1
  Gain/1 -> steerCmd/1
  Curvature/1 -> ?
  CurrVelocity/1 -> Lateral Controller Stanley/3
  RefPoses/1 -> Demux/1, Lateral Controller Stanley/1
  Pose/1 -> Pure Pursuit Controller1/1(Pose)
  Lateral Controller Stanley/1 -> Unit Delay/1
  Constant/1 -> Lateral Controller Stanley/4
  Demux1/2 -> Scope2/2
  Demux/2 -> Scope2/1
  Gain2/1 -> Gain/1
  Waypoints/1 -> Pure Pursuit Controller1/2(Waypoints)

== system vehicle_hostmodel_2022b_v10/Controllers/Longitudinal Controllers ==
  Curr Velocity : Inport
  Relative velocity : Inport  Port=2
  Relative distance : Inport  Port=3
  Time gap : Inport  Port=4
  Set velocity : Inport  Port=5
  CurrVel : Inport  Port=6
  Adaptive Cruise Control System : mpcadaslib/Adaptive Cruise Control System  Commented=on  EgoModel=tf(1,[0.5,1,0])  InitialEgoVelocity=0  DefaultSpacing=WB+2  MaxVelocity=50  MinAcceleration=-40  amin_ext=off  MaxAcceleration=40  amax_ext=off  Ts=0.1  PredictionHorizon=10  ControllerBehavior=1.0  suboptimal=off  maxiter=10  datatypeopt=double  optmode=off  trackmode=off
  Constant : Constant
  Constant3 : Constant  Value=0
  Longitudinal Controller Stanley : drivingvehiclecontroller/Longitudinal Controller Stanley  Commented=on  Kp=5  Ki=2  SampleTime=0.05  MaxAcceleration=40  MaxDeceleration=40
  Longitudinal acceleration : Outport
  AccelCmd : Outport  Port=2
  DecelCmd : Outport  Port=3
  wires:
  Set velocity/1 -> Longitudinal Controller Stanley/1, Adaptive Cruise Control System/1
  Constant3/1 -> Longitudinal Controller Stanley/4
  Curr Velocity/1 -> Adaptive Cruise Control System/3
  CurrVel/1 -> Longitudinal Controller Stanley/2
  Longitudinal Controller Stanley/1 -> AccelCmd/1
  Longitudinal Controller Stanley/2 -> DecelCmd/1
  Relative velocity/1 -> Adaptive Cruise Control System/5
  Relative distance/1 -> Adaptive Cruise Control System/4
  Adaptive Cruise Control System/1 -> Longitudinal acceleration/1
  Time gap/1 -> Adaptive Cruise Control System/2
  Constant/1 -> Longitudinal Controller Stanley/3

== system vehicle_hostmodel_2022b_v10/Controllers/Subsystem1 ==
  VehFdbk : Inport
  Bus Selector : BusSelector  OutputSignals=InertFrm.Cg.Disp.X,InertFrm.Cg.Disp.Y,InertFrm.Cg.Ang.psi
  Bus Selector1 : BusSelector  Commented=on  OutputSignals=InertFrm.Cg.Disp.X,InertFrm.Cg.Disp.Y,InertFrm.Cg.Disp.Z
  Gain1 : Gain  Gain=180/pi
  Mux : Mux  Inputs=3
  Mux1 : Mux  Commented=on  Inputs=3
  Mux2 : Mux  Inputs=3
  Transpose : Math  Operator=transpose  SignedPower=on
  Transpose1 : Math  Commented=on  Operator=transpose  SignedPower=on
  Transpose2 : Math  Operator=transpose  SignedPower=on
  pose : Outport
  PPpose : Outport  Port=2
  wires:
  Mux/1 -> Transpose/1
  VehFdbk/1 -> Bus Selector1/1, Bus Selector/1
  Gain1/1 -> Mux/3
  Transpose/1 -> pose/1
  Bus Selector/3 -> Mux2/3, Gain1/1  "<psi>"
  Bus Selector1/1 -> Mux1/1  "<X>"
  Bus Selector1/2 -> Mux1/2  "<Y>"
  Bus Selector1/3 -> Mux1/3  "<Z>"
  Mux1/1 -> Transpose1/1
  Mux2/1 -> Transpose2/1
  Transpose2/1 -> PPpose/1
  Bus Selector/2 -> Mux/2, Mux2/2  "<Y>"
  Bus Selector/1 -> Mux/1, Mux2/1  "<X>"

== system vehicle_hostmodel_2022b_v10/Controllers/Subsystem2 ==
  ACCaccel_cmd : Inport
  LCaccel_cmd : Inport  Port=2
  LCdeccel_cmd : Inport  Port=3
  ACC : Inport  Port=4
  CurrVelocity : Inport  Port=5
  Relative Distance : Inport  Port=6
  Braking : Inport  Port=7
  CurrAccel : Inport  Port=8
  Constant : Constant  Value=0
  MATLAB Function : MATLAB Function  Commented=on  TreatAsAtomicUnit=on
  Subsystem : Subsystem
  Subsystem1 : Subsystem
  Switch{,1..3} (4 alike) : Switch  Commented=on  Criteria=u2 > Threshold  SaturateOnIntegerOverflow=off  InputSameDT=off
  TorgueCm : Outport
  BrakeCm : Outport  Port=2
  wires:
  Subsystem1/2(brake_cm) -> BrakeCm/1, Switch2/3
  Subsystem1/1(torque_cm) -> TorgueCm/1, Switch3/3
  ACCaccel_cmd/1 -> MATLAB Function/1(u)
  ACC/1 -> Switch/2
  MATLAB Function/1(accel) -> Switch/1
  LCaccel_cmd/1 -> Subsystem1/1(acc_cmd), Switch/3
  LCdeccel_cmd/1 -> Subsystem1/2(decc_cmd), Switch1/3
  MATLAB Function/2(decel) -> Switch1/1
  Constant/1 -> Switch3/1
  Braking/1 -> Switch3/2, Switch2/2, Subsystem/4("Braking ")
  CurrVelocity/1 -> Subsystem/1(CurrVelocity)
  Relative Distance/1 -> Subsystem/2(Relative Distance)
  Subsystem/1(BrakeCm) -> Switch2/1
  CurrAccel/1 -> Subsystem/3(CurrAccel)

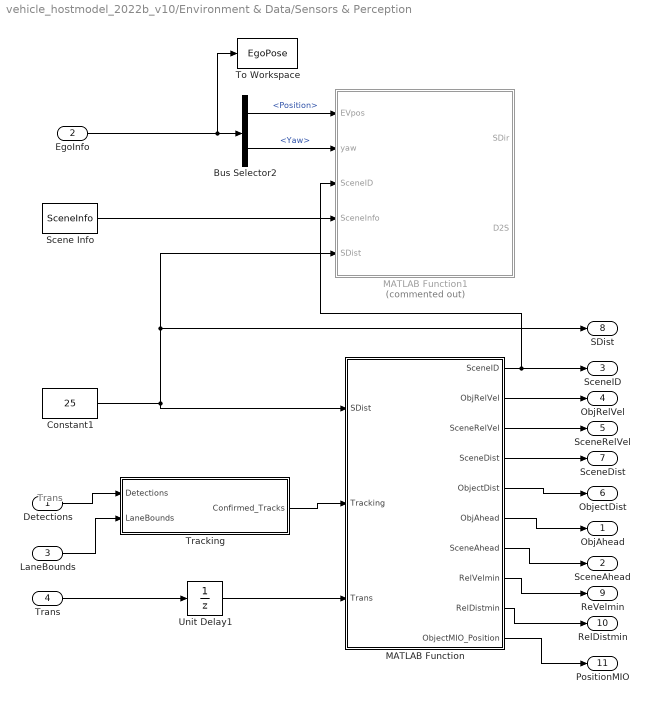
== system vehicle_hostmodel_2022b_v10/Environment & Data/Sensors & Perception ==
  note: Trans
  Detections : Inport
  EgoInfo : Inport  Port=2
  LaneBounds : Inport  Port=3
  Trans : Inport  Port=4
  Bus Selector2 : BusSelector  OutputSignals=Position,Yaw
  Constant1 : Constant  Value=25
  MATLAB Function : MATLAB Function  TreatAsAtomicUnit=on
  MATLAB Function1 : MATLAB Function  Commented=on  TreatAsAtomicUnit=on
  Scene Info : Constant  Value=SceneInfo  VectorParams1D=off
  To Workspace : ToWorkspace  VariableName=EgoPose  SaveFormat=Timeseries  SampleTime=-1
  Tracking : Subsystem
  Unit Delay1 : UnitDelay  SampleTime=0.05  HasFrameUpgradeWarning=on
  ObjAhead : Outport
  SceneAhead : Outport  Port=2
  SceneID : Outport  Port=3
  ObjRelVel : Outport  Port=4
  SceneRelVel : Outport  Port=5
  ObjectDist : Outport  Port=6
  SceneDist : Outport  Port=7
  SDist : Outport  Port=8
  ReVelmin : Outport  Port=9
  RelDistmin : Outport  Port=10
  PositionMIO : Outport  Port=11
  wires:
  MATLAB Function/6(ObjAhead) -> ObjAhead/1
  MATLAB Function/5(ObjectDist) -> ObjectDist/1
  MATLAB Function/7(SceneAhead) -> SceneAhead/1
  MATLAB Function/2(ObjRelVel) -> ObjRelVel/1
  EgoInfo/1 -> To Workspace/1, Bus Selector2/1
  Bus Selector2/1 -> MATLAB Function1/1(EVpos)  "<Position>"
  Detections/1 -> Tracking/1(Detections)
  Scene Info/1 -> MATLAB Function1/4(SceneInfo)
  Bus Selector2/2 -> MATLAB Function1/2(yaw)  "<Yaw>"
  Tracking/1(Confirmed_Tracks) -> MATLAB Function/2(Tracking)
  Constant1/1 -> MATLAB Function1/5(SDist), SDist/1, MATLAB Function/1(SDist)
  MATLAB Function/1(SceneID) -> MATLAB Function1/3(SceneID), SceneID/1
  MATLAB Function/4(SceneDist) -> SceneDist/1
  MATLAB Function/3(SceneRelVel) -> SceneRelVel/1
  MATLAB Function/8(RelVelmin) -> ReVelmin/1
  MATLAB Function/9(RelDistmin) -> RelDistmin/1
  Trans/1 -> Unit Delay1/1
  Unit Delay1/1 -> MATLAB Function/3(Trans)
  LaneBounds/1 -> Tracking/2(LaneBounds)
  MATLAB Function/10(ObjectMIO_Position) -> PositionMIO/1

== system vehicle_hostmodel_2022b_v10/Environment & Data/Subsystem1 ==
  VehFdbk : Inport
  Bus Selector : BusSelector  OutputSignals=InertFrm.Cg.Disp.X,InertFrm.Cg.Disp.Y,InertFrm.Cg.Ang.psi
  Gain1 : Gain  Gain=180/pi
  Mux : Mux  Inputs=3
  Transpose : Math  Operator=transpose  SignedPower=on
  pose : Outport
  wires:
  Mux/1 -> Transpose/1
  VehFdbk/1 -> Bus Selector/1
  Gain1/1 -> Mux/3
  Transpose/1 -> pose/1
  Bus Selector/3 -> Gain1/1  "<psi>"
  Bus Selector/2 -> Mux/2  "<Y>"
  Bus Selector/1 -> Mux/1  "<X>"

== system vehicle_hostmodel_2022b_v10/Environment & Data/Visualisation & Data ==
  note: Load Scenario
  note: Traffic Lights and Stop Signs
  EgoVehStates : Inport
  EgoVelocity : Inport  Port=2
  Ego Acceleration : Inport  Port=3
  Ego Position : Inport  Port=4
  EgoInfo : Inport  Port=5
  Bus Selector : BusSelector  OutputSignals=Actors
  Display : Display
  Display3 : Display
  Lights and Signs ID : Subsystem
  "Positions and States " : Subsystem
  Scenario Reader : drivingscenarioandsensors/Scenario Reader  ScenarioSource=From file  ScenarioFileName=/Users/rahulmathias/Desktop/Autodrive Challenge_2/planningControl-Simulation-Gitcheck/scenarios/Longroadtest.mat  ScenarioVariableName=scenario  OutputCoordinateSystem=Vehicle coordinates  EgoVehicleSource=Input port  EgoVehicleActorID=1  OrientVehiclesOnRoad=on  OutputEgoVehiclePose=on  OutputEgoVehicleState=off  SampleTime=Ts  LaneBoundaryOutput=All lane boundaries  LaneBoundaryDistance=0:0.5:9.5  LaneBoundaryLocation=Center of lane markings  BusNameSource=Auto  BusName=BusActors  BusNumActorsSource=Scenario  BusNumActors=100  BusName2Source=Auto  BusName2=BusLaneBoundaries  BusNumLaneBoundariesSource=Scenario  BusNumLaneBoundaries=10  BusName3Source=Auto  BusName3=BusEgoActor  BusName4Source=Auto  BusName4=BusEgoState  ShowCoordinateLabels=on  SimulateUsing=Interpreted execution
  To Workspace : ToWorkspace  VariableName=SimVel  SampleTime=-1
      settings: Save2DSignal=2-D array (concatenate along first dimension)
  To Workspace1 : ToWorkspace  VariableName=actors  SaveFormat=Timeseries  SampleTime=-1
  To Workspace9 : ToWorkspace  VariableName=SimPos  SampleTime=-1
      settings: Save2DSignal=2-D array (concatenate along first dimension)
  Vehicle To World : drivingscenarioandsensors/Vehicle To World  BusNameSource=Auto  BusName=BusVehicleToWorldActors  SimulateUsing=Interpreted execution
  Visualization : Subsystem
  Actors_VehCoords : Outport
  TL_poses : Outport  Port=2
  actorsinfo : Outport  Port=3
  LaneBounds : Outport  Port=4
  wires:
  Vehicle To World/1 -> To Workspace1/1, actorsinfo/1, Bus Selector/1, Visualization/2(Actors)
  EgoVelocity/1 -> To Workspace/1, Display/1
  Scenario Reader/1 -> Vehicle To World/1, Actors_VehCoords/1
  "Positions and States "/1(TL_poses) -> TL_poses/1, Visualization/1(TL1_poses)
  Lights and Signs ID/1(TL) -> "Positions and States "/2(TL_id)
  Lights and Signs ID/2(Stop_Sign) -> "Positions and States "/3(ss_State)
  "Positions and States "/2(ss_poses) -> Visualization/4(ss1_poses)
  Ego Acceleration/1 -> Display3/1
  Ego Position/1 -> To Workspace9/1
  EgoInfo/1 -> Visualization/3(EgoInfo)
  EgoVehStates/1 -> Vehicle To World/2, Scenario Reader/1
  Bus Selector/1 -> "Positions and States "/1(<Actors>)  "<Actors>"
  Scenario Reader/2 -> LaneBounds/1

== system vehicle_hostmodel_2022b_v10/Reference Data/Theta ==
  note: 1) Add Subsystem or Model blocks as valid variant choices.
      | 2) You cannot connect blocks at this level. At simulation, connectivity is automatically
      | determined, based on the active variant and port name matching.
  y : Inport
  x : Inport  Port=2
  dis : Inport  Port=3
  thetaBlocks : Subsystem  VariantControl=thetaSimulinkBlock
  thetaLt : Subsystem  VariantControl=thetaLookUpTable
  theta : Outport

== system vehicle_hostmodel_2022b_v10/Reference Data1/Subsystem ==
  In1 : Inport
  Enable : EnablePort
  Step : Step
  Step1 : Step  Time=10
  Sum : Sum  Inputs=|+-
  Out1 : Outport
  wires:
  Sum/1 -> Out1/1
  Step/1 -> Sum/1
  Step1/1 -> Sum/2

== system vehicle_hostmodel_2022b_v10/Reference Data1/Subsystem1 ==
  Integrator : Inport
  enable : Inport  Port=2
  Display : Display
  Subsystem2 : Subsystem
  Subsystem3 : Subsystem
  Switch : Switch  Threshold=1  SaturateOnIntegerOverflow=off  InputSameDT=off
  Ref pose : Outport
  wires:
  enable/1 -> Switch/2
  Integrator/1 -> Subsystem2/1(Integrator), Subsystem3/2(integrator)
  Subsystem2/1(RefPose) -> Display/1, Switch/3
  Subsystem3/1(RefPose) -> Switch/1
  Switch/1 -> Ref pose/1
